simulink model "INTMLStateCtrl"  (R2018b)
settings: Solver=FixedStepDiscrete  StartTime=0.0  StopTime=10.0  FixedStep=0.01  RelTol=1e-3
libraries: StateCtrlLib x1
settings Model: Creator=sn2xws  LastModifiedBy=sn2xws
settings DataIOCC: SaveFormat=StructureWithTime
settings OptimizationCC: DefaultParameterBehavior=Inlined  EnhancedBackFolding=on  PassReuseOutputArgsAs=Individual arguments  ZeroExternalMemoryAtStartup=off  ZeroInternalMemoryAtStartup=off  OptimizeBlockOrder=speed  DifferentSizesBufferReuse=on  OptimizationCustomize=off
settings DebuggingCC: ParameterTunabilityLossMsg=error
settings ModelReferenceCC: ModelReferenceNumInstancesAllowed=Single
settings SFSimCC: MATLABDynamicMemAlloc=off
settings RTWCC: SystemTargetFile=autosar.tlc  GenCodeOnly=on  TemplateMakefile=ert_default_tmf  Description=AUTOSAR  GenerateReport=on  IncludeHyperlinkInReport=on  LaunchReport=on  GenerateTraceInfo=on  GenerateTraceReport=on  GenerateTraceReportSl=on  GenerateTraceReportSf=on  GenerateTraceReportEml=on
settings CodeAppCC: ForceParamTrailComments=on  IgnoreCustomStorageClasses=off  OperatorAnnotations=on  SimulinkDataObjDesc=on  SFDataObjDesc=on  InsertBlockDesc=on
settings STFCustomTargetCC: TargetLangStandard=C99 (ISO)  MultiwordLength=256  ParMdlRefBuildCompliant=on  CompOptLevelCompliant=on  IncludeMdlTerminateFcn=off  CombineOutputUpdateFcns=on  SuppressErrorStatus=on  ERTCustomFileBanners=on  SupportNonFinite=off  SupportComplex=off  SupportContinuousTime=off  SupportNonInlinedSFcns=off  RemoveResetFunc=on  MATLABClassNameForMDSCustomization=Simulink.SoftwareTarget.ERTCustomization  AutosarCompliant=on  UseToolchainInfoCompliant=on  LookupTableObjectStructAxisOrder=2,1,3,4,...  LUTObjectStructOrderEvenSpacing=Size,Table,Breakpoints  SystemTargetFile=autosar.tlc
settings ERTTargetCC: TargetLangStandard=C99 (ISO)  ConcurrentExecutionCompliant=off  IncludeMdlTerminateFcn=off  SuppressErrorStatus=on  SupportNonFinite=off  SupportComplex=off  ModelStepFunctionPrototypeControlCompliant=off  CPPClassGenCompliant=off  AutosarCompliant=on  LookupTableObjectStructAxisOrder=2,1,3,4,...  LUTObjectStructOrderEvenSpacing=Size,Table,Breakpoints  InlinedParameterPlacement=NonHierarchical  ERTCustomFileTemplate=example_file_process.tlc

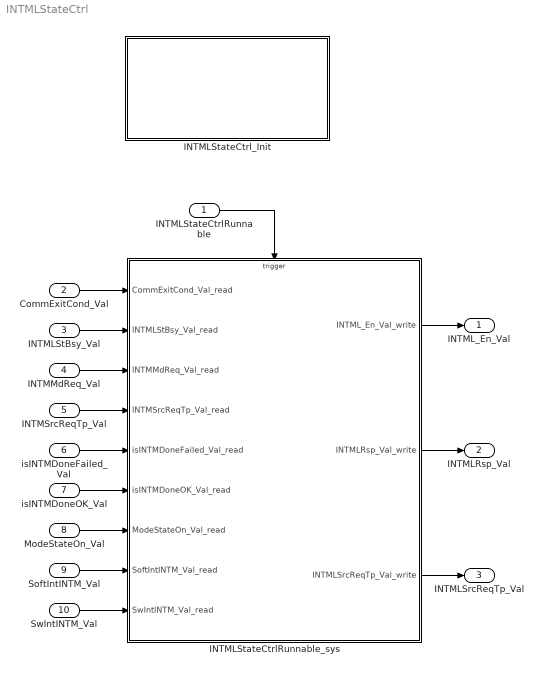
== system INTMLStateCtrl ==
  INTMLStateCtrlRunnable : Inport  SampleTime=0.01  OutputFunctionCall=on
  CommExitCond_Val : Inport  Port=2  OutDataTypeStr=boolean  PortDimensions=1
  INTMLStBsy_Val : Inport  Port=3  OutDataTypeStr=boolean  PortDimensions=1
  INTMMdReq_Val : Inport  Port=4  OutDataTypeStr=boolean  PortDimensions=1
  INTMSrcReqTp_Val : Inport  Port=5  OutDataTypeStr=Enum: SrcReqTp1  PortDimensions=1
  isINTMDoneFailed_Val : Inport  Port=6  OutDataTypeStr=boolean  PortDimensions=1
  isINTMDoneOK_Val : Inport  Port=7  OutDataTypeStr=boolean  PortDimensions=1
  ModeStateOn_Val : Inport  Port=8  OutDataTypeStr=boolean  PortDimensions=1
  SoftIntINTM_Val : Inport  Port=9  OutDataTypeStr=IntEnable  PortDimensions=1
  SwIntINTM_Val : Inport  Port=10  OutDataTypeStr=IntEnable  PortDimensions=1
  INTMLStateCtrlRunnable_sys : Subsystem
  INTMLStateCtrl_Init : Subsystem
  INTML_En_Val : Outport  OutDataTypeStr=boolean  PortDimensions=1
  INTMLRsp_Val : Outport  Port=2  OutDataTypeStr=Enum: MdRspLocal1  PortDimensions=1
  INTMLSrcReqTp_Val : Outport  Port=3  OutDataTypeStr=Enum: SrcReqTp1  PortDimensions=1
  wires:
  CommExitCond_Val/1 -> INTMLStateCtrlRunnable_sys/1(CommExitCond_Val_read)
  INTMLStBsy_Val/1 -> INTMLStateCtrlRunnable_sys/2(INTMLStBsy_Val_read)
  INTMMdReq_Val/1 -> INTMLStateCtrlRunnable_sys/3(INTMMdReq_Val_read)
  INTMSrcReqTp_Val/1 -> INTMLStateCtrlRunnable_sys/4(INTMSrcReqTp_Val_read)
  isINTMDoneFailed_Val/1 -> INTMLStateCtrlRunnable_sys/5(isINTMDoneFailed_Val_read)
  isINTMDoneOK_Val/1 -> INTMLStateCtrlRunnable_sys/6(isINTMDoneOK_Val_read)
  ModeStateOn_Val/1 -> INTMLStateCtrlRunnable_sys/7(ModeStateOn_Val_read)
  SoftIntINTM_Val/1 -> INTMLStateCtrlRunnable_sys/8(SoftIntINTM_Val_read)
  SwIntINTM_Val/1 -> INTMLStateCtrlRunnable_sys/9(SwIntINTM_Val_read)
  INTMLStateCtrlRunnable_sys/1(INTML_En_Val_write) -> INTML_En_Val/1
  INTMLStateCtrlRunnable_sys/2(INTMLRsp_Val_write) -> INTMLRsp_Val/1
  INTMLStateCtrlRunnable_sys/3(INTMLSrcReqTp_Val_write) -> INTMLSrcReqTp_Val/1
  INTMLStateCtrlRunnable/1 -> INTMLStateCtrlRunnable_sys/Trigger

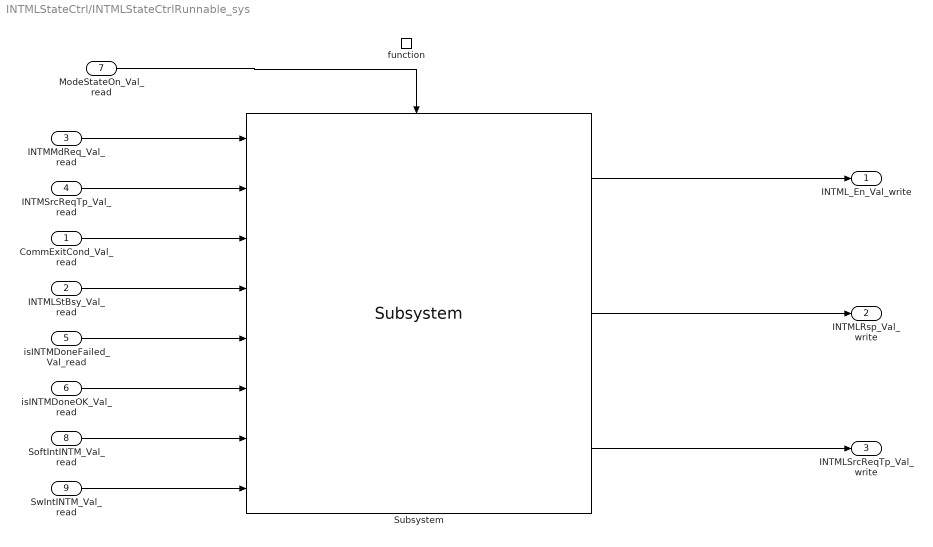
== system INTMLStateCtrl/INTMLStateCtrlRunnable_sys ==
  CommExitCond_Val_read : Inport
  INTMLStBsy_Val_read : Inport  Port=2
  INTMMdReq_Val_read : Inport  Port=3
  INTMSrcReqTp_Val_read : Inport  Port=4
  isINTMDoneFailed_Val_read : Inport  Port=5
  isINTMDoneOK_Val_read : Inport  Port=6
  ModeStateOn_Val_read : Inport  Port=7
  SoftIntINTM_Val_read : Inport  Port=8  OutDataTypeStr=IntEnable
  SwIntINTM_Val_read : Inport  Port=9  OutDataTypeStr=IntEnable
  function : TriggerPort  TriggerType=function-call  VariantControl=(inherit)  SampleTimeType=periodic  SampleTime=-1
  Subsystem : StateCtrlLib/Subsystem  SystemSampleTime=-1
  INTML_En_Val_write : Outport
      settings: EnsureOutportIsVirtual=on
  INTMLRsp_Val_write : Outport  Port=2
      settings: EnsureOutportIsVirtual=on
  INTMLSrcReqTp_Val_write : Outport  Port=3
      settings: EnsureOutportIsVirtual=on
  wires:
  Subsystem/1 -> INTML_En_Val_write/1
  Subsystem/2 -> INTMLRsp_Val_write/1
  Subsystem/3 -> INTMLSrcReqTp_Val_write/1
  ModeStateOn_Val_read/1 -> Subsystem/Enable
  INTMLStBsy_Val_read/1 -> Subsystem/4
  CommExitCond_Val_read/1 -> Subsystem/3
  isINTMDoneFailed_Val_read/1 -> Subsystem/5
  isINTMDoneOK_Val_read/1 -> Subsystem/6
  SoftIntINTM_Val_read/1 -> Subsystem/7
  SwIntINTM_Val_read/1 -> Subsystem/8
  INTMMdReq_Val_read/1 -> Subsystem/1
  INTMSrcReqTp_Val_read/1 -> Subsystem/2

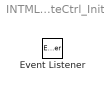
== system INTMLStateCtrl/INTMLStateCtrl_Init ==
  Event Listener : EventListener  EventName=reset
